simulink model "part5_observer_windows_target"  (R2014a)
settings: Solver=ode1  StartTime=0.0  StopTime=100  FixedStep=0.005  RelTol=1e-3
undefined symbols (not defined in the file): A_0, B_0, C_0, D_0
libraries: c6xlib x2, fricblocks x1
Description:
  | Real-Time Van der Pol Simulation
  | 
  | This demonstration shows a real-time version of the Simulink(R) Van der Pol
  | simulation demo. This model does not need any external signals, so it does
  | not need any data acquisition hardware or driver. This makes the model ideal
  | for first experiments with Real-Time Windows Target(TM), without need to
  | worry about proper I/O hardware configuration.
  | 
  | How to run this demo:
  | 
  |   1. Build the model using Tools -> Real-Time Workshop -> Build Model.
  |   2. Connect to the real-time code using Simulation -> Connect to target.
  |   3. Start the real-time execution using Simulation -> Start real-time code.
settings Model: SimulationMode=external  ExtModeTrigDuration=50000  Creator=Houska  LastModifiedBy=mmroman2
settings DataIOCC: SignalLoggingSaveFormat=ModelDataLogs  SignalLoggingName=logsOut
settings OptimizationCC: ExpressionDepthLimit=2147483647  InitFltsAndDblsToZero=on  EfficientMapNaN2IntZero=off
settings DebuggingCC: UnderspecifiedInitializationDetection=Classic  SignalResolutionControl=TryResolveAllWithWarning  SolverPrmCheckMsg=none  FcnCallInpInsideContextMsg=UseLocalSettings  StateNameClashWarn=warning
settings HardwareCC: ProdIntDivRoundTo=Zero  ProdEndianess=LittleEndian  ProdHWDeviceType=32-bit Real-Time Windows Target
settings RTWCC: SystemTargetFile=rtwin.tlc  TemplateMakefile=rtwin.tmf  Description=Real-Time Windows Target  ProcessScript=rtwin_make_rtw_hook
settings RTWinTargetCC: TargetLibSuffix=_rtwin.lib  TargetPreCompLibLocation=C:\MATLABR2014a\toolbox\rtw\targets\rtwin\lib\win64

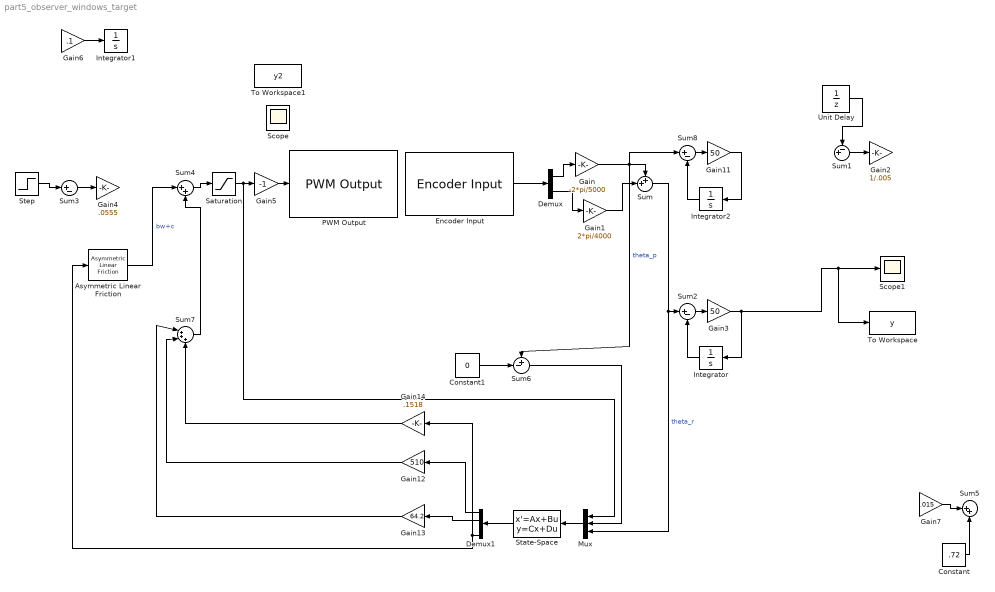
== system part5_observer_windows_target ==
  Asymmetric Linear Friction : fricblocks/Asymmetric  Linear Friction  intercept1=.72  intercept2=-.76  slope1=.01  slope2=.01
  Constant : Constant  Value=.72
  Constant1 : Constant  Value=0
  Demux : Demux  Outputs=2
  Demux1 : Demux
  Encoder Input : c6xlib/Encoder Input  baseAddr=0x378  channels=[0 1]  sampleTime=str2num(get_param(bdroot, 'FixedStep'))
  Gain : Gain  Gain=-2*pi/5000
  Gain1 : Gain  Gain=2*pi/4000
  Gain11 : Gain  Gain=50
  Gain12 : Gain  Gain=510
  Gain13 : Gain  Gain=64.2
  Gain14 : Gain  Gain=.1518
  Gain2 : Gain  Gain=1/.005
  Gain3 : Gain  Gain=50
  Gain4 : Gain  Gain=.0555
  Gain5 : Gain  Gain=-1
  Gain6 : Gain  Gain=.1
  Gain7 : Gain  Gain=.015
  Integrator : Integrator
  Integrator1 : Integrator
  Integrator2 : Integrator
  Mux : Mux  Inputs=3
  PWM Output : c6xlib/PWM Output  baseAddr=0x378  channels=0  initialOutputs=0  finalOutputs=0  sampleTime=str2num(get_param(bdroot, 'FixedStep'))
  Saturation : Saturate  UpperLimit=10  LowerLimit=-10
  Scope : Scope
  Scope1 : Scope
      settings: YMin=0  YMax=95
  State-Space : StateSpace  A=A_0  B=B_0  C=C_0  D=D_0  X0=0
  Step : Step  Time=0  After=-100  SampleTime=0
  Sum : Sum  Inputs=++|
  Sum1 : Sum  Inputs=-+|
  Sum2 : Sum  Inputs=|+-
  Sum3 : Sum  Inputs=|+-
  Sum4 : Sum  Inputs=|++
  Sum5 : Sum  Inputs=|++
  Sum6 : Sum  Inputs=+-|
  Sum7 : Sum  Inputs=|+++
  Sum8 : Sum  Inputs=|+-
  To Workspace : ToWorkspace  VariableName=y  SampleTime=-1
  To Workspace1 : ToWorkspace  VariableName=y2  SampleTime=-1
  Unit Delay : UnitDelay  SampleTime=-1
  wires:
  Demux/2 -> Gain1/1
  Demux/1 -> Gain/1
  Encoder Input/1 -> Demux/1
  Gain/1 -> Sum6/1, Sum8/1, Sum/1  "theta_p"
  Gain1/1 -> Sum/2
  Sum/1 -> Mux/3, Sum2/1  "theta_r"
  Unit Delay/1 -> Sum1/1
  Sum1/1 -> Gain2/1
  Integrator/1 -> Sum2/2
  Sum2/1 -> Gain3/1
  Step/1 -> Sum3/1
  Gain3/1 -> To Workspace/1, Scope1/1, Integrator/1
  Saturation/1 -> Mux/1, Gain5/1
  Gain5/1 -> PWM Output/1
  Sum3/1 -> Gain4/1
  Gain6/1 -> Integrator1/1
  Gain7/1 -> Sum5/1
  Constant/1 -> Sum5/2
  Gain11/1 -> Integrator2/1
  Integrator2/1 -> Sum8/2
  Sum8/1 -> Gain11/1
  Sum7/1 -> Sum4/2
  Sum4/1 -> Saturation/1
  Constant1/1 -> Sum6/2
  Asymmetric Linear Friction/1 -> Sum4/1  "bw+c"
  Gain12/1 -> Sum7/2
  Gain13/1 -> Sum7/1
  Gain14/1 -> Sum7/3
  Mux/1 -> State-Space/1
  State-Space/1 -> Demux1/1
  Demux1/1 -> Gain12/1
  Demux1/2 -> Gain13/1
  Demux1/4 -> Gain14/1, Asymmetric Linear Friction/1
  Sum6/1 -> Mux/2
